simulink model "TankPID_f13"  (R2013b)
settings: Solver=ode5  StartTime=0.0  StopTime=inf  FixedStep=0.1  RelTol=1e-3
undefined symbols (not defined in the file): MIO, National_Instruments, PCI
libraries: rtwinlib x3
settings Model: SimulationMode=external  Creator=melab  LastModifiedBy=melab
settings HardwareCC: ProdIntDivRoundTo=Zero  ProdEndianess=LittleEndian  ProdHWDeviceType=Generic->32-bit x86 compatible
settings RTWCC: SystemTargetFile=rtwin.tlc  TemplateMakefile=rtwin.tmf  Description=Real-Time Windows Target  ProcessScript=rtwin_make_rtw_hook  Toolchain=LCC-win32 v2.4.1 | gmake (32-bit Windows)  RTWCompilerOptimization=On
settings CodeAppCC: MaxIdLength=95
settings RTWinTargetCC: TargetLibSuffix=_rtwin.lib  TargetPreCompLibLocation=C:\Program Files\MATLAB\R2013b\toolbox\rtw\targets\rtwin\lib\win32  CodeReplacementLibrary=ANSI_C  RTWinDir=C:/PROGRA~1/MATLAB/R2013b/toolbox/rtw/targets/rtwin  TargetArch=win32

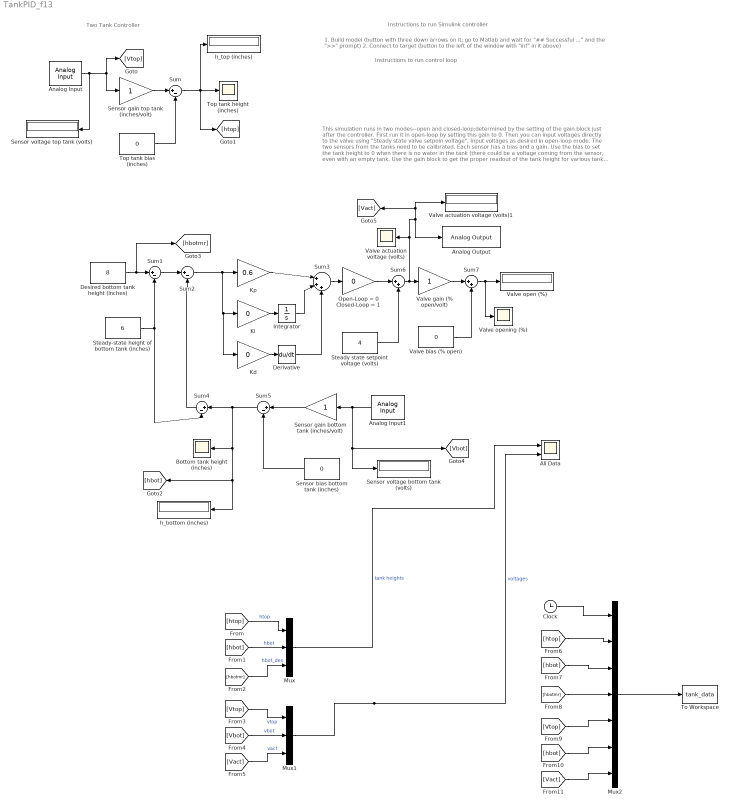
== system TankPID_f13 ==
  note: Two Tank Controller
  note: This simulation runs in two modes--open and closed-loop;determined by the setting of the gain block just after
      | the controller.  First run it in open-loop by setting this gain to 0.  Then you can input voltages directly to the valve using
      | "Steady state valve setpoin voltage".  Input voltages as desired in open-loop mode.
      |
      | The two sensors from the tanks need to be calibrated.  Each sensor has a bias and a gain.  Use the bias to set the
      | tank height to 0 when there is no water in the tank (there could be a voltage coming from the sensor, even with an
      | empty tank.  Use the gain block to get the proper readout of the tank height for various tank heights.
      |
      | Likewise, the valve %-opening read-out can be calibrated.  This gives a rough estimate of the valve position.  But
      | it is just working from the input voltage signal to the valve, so it should not be fully trusted.
      |
      | Once you get everything calibrated correctly and the system running at a steady state, you can run the loop in  closed-loop.
      | The loop works on deviations from your desired or design steady state.  Make sure that you first put the steady state
      | height of the bottom tank in "Steady state height of bottom tank".  Set also "Desired height of bottom tank" to this same value,
      | the beginning AND the end values.  Then the loop should run at this level until you change something.
  note: 1. Build model (button with three down arrows on it; go to Matlab and wait for "## Successful ..." and the ">>" prompt)
      | 2. Connect to target (button to the left of the window with "inf" in it above)
  note: Instructions to run Simulink controller
  note: Instructions to run control loop
  All Data : Scope  NumInputPorts=2
      settings: TickLabels=on  ShowLegends=on  YMin=6~4  YMax=8~6.75  SaveName=ScopeData4
  Analog Input : rtwinlib/Analog Input  SampleTime=0.1  MaxMissedTicks=10  ShowMissedTicks=off  YieldWhenWaiting=off  DrvName=National_Instruments/PCI-MIO-16E-4  DrvAddress=4294967295  DrvOptions=[0 0 0 0 0 0]  Channels=4  RangeMode=1  VoltRange=1  DataType=1
      settings: AttributesFormatString=National Instruments\nPCI-MIO-16E-4 [auto]
  Analog Input1 : rtwinlib/Analog Input  SampleTime=0.1  MaxMissedTicks=10  ShowMissedTicks=off  YieldWhenWaiting=off  DrvName=National_Instruments/PCI-MIO-16E-4  DrvAddress=4294967295  DrvOptions=[0 0 0 0 0 0]  Channels=5  RangeMode=1  VoltRange=1  DataType=1
      settings: AttributesFormatString=National Instruments\nPCI-MIO-16E-4 [auto]
  Analog Output : rtwinlib/Analog Output  SampleTime=0.1  MaxMissedTicks=10  ShowMissedTicks=off  YieldWhenWaiting=off  DrvName=National_Instruments/PCI-MIO-16E-4  DrvAddress=4294967295  DrvOptions=[0 0 0 0 0 0]  Channels=1  RangeMode=1  VoltRange=1  InitialValue=[]  FinalValue=[]
      settings: AttributesFormatString=National Instruments\nPCI-MIO-16E-4 [auto]
  Bottom tank height (inches) : Scope
      settings: TimeRange=500  YMin=6.2  YMax=6.5  SaveName=ScopeData2
  Clock : Clock
  Derivative : Derivative
  Desired bottom tank height (inches) : Constant  Value=8
  Integrator : Integrator
  Kd : Gain  Gain=0
  Ki : Gain  Gain=0
  Kp : Gain  Gain=0.6
  Mux : Mux  Inputs=3
  Mux1 : Mux  Inputs=3
  Mux2 : Mux  Inputs=7
  Open-Loop = 0 Closed-Loop = 1 : Gain  Gain=0
  Sensor bias bottom tank (inches) : Constant  Value=0
  Sensor gain top tank (inches/volt) : Gain
  Sensor gain bottom tank (inches/volt) : Gain
  Sensor voltage bottom tank (volts) : Display
  Sensor voltage top tank (volts) : Display
  Steady state setpoint voltage (volts) : Constant  Value=4
  "Steady-state height of bottom tank (inches) " : Constant  Value=6
  Sum{,1..2,4..5} (5 alike) : Sum  Inputs=|+-
  Sum3 : Sum  Inputs=|+++
  Sum6 : Sum  Inputs=|++
  Sum7 : Sum  Inputs=|++
  To Workspace : ToWorkspace  VariableName=tank_data  SampleTime=-1
  Top tank height (inches) : Scope
      settings: TimeRange=500  YMin=6  YMax=10
  Top tank bias (inches) : Constant  Value=0
  Valve actuation voltage (volts) : Scope
      settings: TimeRange=500  YMin=6  YMax=10  SaveName=ScopeData3
  "Valve actuation voltage (volts)1 " : Display
  Valve bias (% open) : Constant  Value=0
  Valve gain (% open/volt) : Gain
  Valve open (%) : Display
  Valve opening (%) : Scope
      settings: TimeRange=500  YMin=2.67125  YMax=2.6745
  h_bottom (inches) : Display
  h_top (inches) : Display
  wires:
  Top tank bias (inches)/1 -> Sum/2
  Analog Input/1 -> Sensor voltage top tank (volts)/1, Sensor gain top tank (inches/volt)/1, [Vtop]
  Sensor gain top tank (inches/volt)/1 -> Sum/1
  Sum/1 -> h_top (inches)/1, [htop], Top tank height (inches)/1
  Kp/1 -> Sum3/1
  Ki/1 -> Integrator/1
  Integrator/1 -> Sum3/2
  Kd/1 -> Derivative/1
  Derivative/1 -> Sum3/3
  Desired bottom tank height (inches)/1 -> [hbotmr], Sum1/1
  Sum1/1 -> Sum2/1
  Sum2/1 -> Kp/1, Kd/1, Ki/1
  "Steady-state height of bottom tank (inches) "/1 -> Sum4/2, Sum1/2
  Sum4/1 -> Sum2/2
  Analog Input1/1 -> [Vbot], Sensor voltage bottom tank (volts)/1, Sensor gain bottom tank (inches/volt)/1
  Sensor gain bottom tank (inches/volt)/1 -> Sum5/1
  Sum5/1 -> h_bottom (inches)/1, [hbot], Bottom tank height (inches)/1, Sum4/1
  Sensor bias bottom tank (inches)/1 -> Sum5/2
  Sum3/1 -> Open-Loop = 0 Closed-Loop = 1/1
  Sum6/1 -> "Valve actuation voltage (volts)1 "/1, [Vact], Analog Output/1, Valve actuation voltage (volts)/1, Valve gain (% open/volt)/1
  Sum7/1 -> Valve open (%)/1, Valve opening (%)/1
  Open-Loop = 0 Closed-Loop = 1/1 -> Sum6/1
  Steady state setpoint voltage (volts)/1 -> Sum6/2
  Valve gain (% open/volt)/1 -> Sum7/1
  Valve bias (% open)/1 -> Sum7/2
  [htop] -> Mux/1  "htop"
  [hbot] -> Mux/2  "hbot"
  Mux1/1 -> All Data/2  "voltages"
  [hbotmr] -> Mux/3  "hbot_des"
  Mux/1 -> All Data/1  "tank heights"
  [Vbot] -> Mux1/2  "vbot"
  [Vact] -> Mux1/3  "vact"
  [Vtop] -> Mux1/1  "vtop"
  [hbotmr] -> Mux2/4
  [Vtop] -> Mux2/5
  Clock/1 -> Mux2/1
  [hbot] -> Mux2/3
  Mux2/1 -> To Workspace/1
  [Vact] -> Mux2/7
  [hbot] -> Mux2/6
  [htop] -> Mux2/2
